simulink model "battery_SimP"  (R2019b)
settings: Solver=ode23tb  StartTime=0.0  StopTime=4000  MaxStep=0.1  RelTol=1e-4  EnableMultiTasking=on
undefined symbols (not defined in the file): Ion, Lithium
libraries: powerlib x2, electricdrivelib x1
Description:
  | Copyright 2008 The MathWorks(TM), Inc.
settings Model: Creator=ac43860  LastModifiedBy=Rene Budich
settings DataIOCC: LimitDataPoints=on  SaveFormat=Array  SignalLoggingSaveFormat=ModelDataLogs  ReturnWorkspaceOutputs=off
settings OptimizationCC: ExpressionDepthLimit=2147483647  InitFltsAndDblsToZero=on  EfficientMapNaN2IntZero=off  LifeSpan=inf
settings DebuggingCC: UnderspecifiedInitializationDetection=Classic  MergeDetectMultiDrivingBlocksExec=none  SignalResolutionControl=TryResolveAllWithWarning  SolverPrmCheckMsg=warning  FcnCallInpInsideContextMsg=warning  StateNameClashWarn=warning  SFUnexpectedBacktrackingDiag=warning  SFNoUnconditionalDefaultTransitionDiag=warning  SFExecutionAtInitializationDiag=none  ArithmeticOperatorsInVariantConditions=warning
settings HardwareCC: ProdBitPerPointer=32  ProdBitPerSizeT=32  ProdBitPerPtrDiffT=32  ProdLargestAtomicFloat=None  ProdIntDivRoundTo=Undefined  ProdEndianess=Unspecified  ProdWordSize=32  ProdHWDeviceType=32-bit Generic
settings ModelReferenceCC: PropagateSignalLabelsOutOfModel=off
settings SFSimCC: SimUseLocalCustomCode=off  CustomCodeUndefinedFunction=UseInterfaceOnly
settings RTWCC: RTWUseLocalCustomCode=off
settings CodeAppCC: StateflowObjectComments=on
settings GRTTargetCC: TargetLangStandard=C89/C90 (ANSI)  CombineOutputUpdateFcns=off  GRTInterface=on
settings ConfigComp: CovMetricSettings=dw  CovHtmlReporting=on  CovSaveCumulativeToWorkspaceVar=on  CovSaveSingleToWorkspaceVar=on

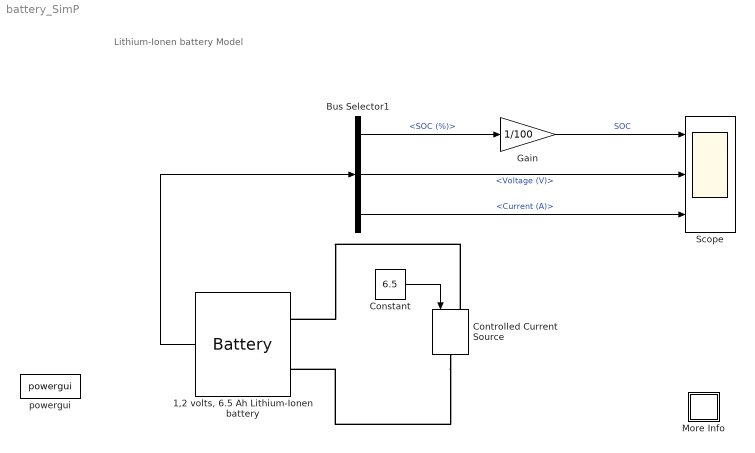
== system battery_SimP ==
  note: Lithium-Ionen battery Model
  "1,2 volts, 6.5 Ah Lithium-Ionen battery " : electricdrivelib/Extra Sources/Battery  BatType=Lithium-Ion  ShowTempParam=off  ThermalPreset=no  ShowAgeParam=off  NomV=1.2  NomQ=6.5  SOC=100  Batt_Tr=30  PresetModel=off  MaxQ=6.825  MinV=0.9  FullV=1.3992  Dis_rate=1.3  R=0.0018462  Normal_OP=5.265  expZone=[1.2696 1.1817]  current=[6.5]  Units=Time  Tci=20  NomT=20  T2=-30  MaxQ2=4.8  FullV2=7.1  Normal_OP2=5.655  expZone2="[6.58           1]"  Rca=0.6  ti=2000  Dp=0  Neq0=0  Tsim=1e6  Ta1=25  Qeol=5.4*0.9  Reol=0.013333*1.2  Char_age=[2.3478, 3]  Dis_age=[2.3478, 10]  N1=1500  N2=10500  N3=1000  N4=1400  Ta2=45  N5=950
      settings: SourceProductName=Simscape Electrical
  Bus Selector1 : BusSelector  OutputSignals=SOC (%),Voltage (V),Current (A)
  Constant : Constant  Value=6.5
  Controlled Current Source : powerlib/Electrical Sources/Controlled Current Source  Initialize=on  Source_Type=AC  Amplitude=0  Phase=0  Frequency=0  Measurements=None
      settings: SourceProductName=Simscape Electrical
  Gain : Gain  Gain=1/100
  More Info : Subsystem
      settings: OpenFcn=showdemo(bdroot(gcb))
      mask Display: disp('?')
  Scope : Scope  NumInputPorts=3
  powergui : powerlib/powergui  SimulationMode=Continuous  SampleTime=0.001  frequency=60  Iterations=50  frequencyindice=0  Pbase=100e6  ErrMax=1e-4  UnitsV=kV  UnitsW=MW  buscounter=0  FunctionMessages=off  echomessages=off  EnableUseOfTLC=off  CurrentSourceSwitches=off  DisableSnubberDevices=off  DisableRonSwitches=off  DisableVfSwitches=off  DisplayEquations=off  AutomaticDiscreteSolvers=off  SolverType=Tustin/Backward Euler (TBE)  Interpol=off  ExternalGateDelay=off  methode=off  Ts=0  x0status=blocks  SPID=off  SwTol=0  HookPort=off  NonlinearTolerance=1e-4  nMaxIteration=100  ContinueOnMaxIteration=off  RestoreLinks=warning  ResistiveCurrentMeasurement=off  Frange=[0:2:500]  Ylog=off  Xlog=on  ShowGrid=off  save=off  variable=ZData  structure=0  ZoomFFT=on  StartTime=0.0  cycles=1  DisplayStyle=1  fundamental=60  FreqAxis=off  MaxFrequency=1000  frequencyindicesteady=1  RmsSteady=1  display=off
      settings: SourceProductName=Simscape Electrical
  wires:
  Constant/1 -> Controlled Current Source/1
  "1,2 volts, 6.5 Ah Lithium-Ionen battery "/1 -> Bus Selector1/1
  Bus Selector1/1 -> Gain/1  "<SOC (%)>"
  Gain/1 -> Scope/1  "SOC"
  Bus Selector1/2 -> Scope/2  "<Voltage (V)>"
  Bus Selector1/3 -> Scope/3  "<Current (A)>"
  connections:
  Controlled Current Source/RConn1 -- "1,2 volts, 6.5 Ah Lithium-Ionen battery "/LConn2
  Controlled Current Source/LConn1 -- "1,2 volts, 6.5 Ah Lithium-Ionen battery "/LConn1

== system battery_SimP/More Info ==
  note: 1) The power system has been discretised with a 20us time step
  note: Notes
  note: H.Blanchette, L.-A. Dessaint (Ecole de technologie superieure, Montreal)
  note: 2) In order to reduce the number of points stored in the scope memory, a decimation factor of 10 is used.
  note: 1) The power sytem has been discretized with a 5us time step. The control system (regulators and braking unit)  uses a 100us time step in
      |      order  to simulate a microcontroller control device.
  note: Notes
  note: This circuit uses the AC1 block of SimPowerSystems library. It models a six-step induction motor drive with a braking chopper for a 3HP AC motor.The induction
      | motor is fed by a voltage source inverter, which is built using the Universal Bridge Block. The DC bus voltage is produced by a thyristor rectifier and regulated using
      | a PI controller in order to maintain a constant volts per hertz ratio. A braking chopper limits the DC bus voltage increase during motor deceleration or when the load
      | torque tends to accelerate the motor. The motor drives a mechanical load characterized by inertia J, friction coefficient B, and load torque TL.
      |
      |  Motor current, speed, and torque signals are available at the output of the block.
  note: Demonstration
  note: Circuit Description
  note: Demonstration of the AC1 Six-Step VSI Induction Motor Drive during speed regulation.
  note: A speed reference step from 0 to 1800 rpm is applied at t = 0. The speed set point doesn't go instantaneously at 1800 rpm but follows the acceleration ramp. The
      | motor reaches steady state at t = 1.3 s.
      |
      | At t =2 s, an accelerating torque is applied on the motor's shaft. You can observe a speed increase. Since the rotor speed is higher than the synchronous speed, the
      | motor is working in the generator mode. The braking energy is transferred to the DC link and the bus voltage tends to increase. However the over voltage activates the
      | braking chopper which causes the voltage to reduce. In this example, the braking resistance is not big enough to avoid a voltage increase but the bus is maintained
      | within tolerable limits.
      |
      | At t = 3 s, the torque applied to the motor's shaft steps from -11 N.m to +11 N.m .You can observe a DC bus voltage and speed drop.  At this point, the DC bus controller
      |  switches from braking to motoring mode.
      |
      | At t = 4 s, the load torque is removed completely and the electromagnetic stabilizes around zero shortly after.
